simulink model "Atabey_Sim"  (R2025b)
settings: Solver=VariableStepAuto  StartTime=0.0  StopTime=simTime  RelTol=1e-3
undefined symbols (not defined in the file or in its folder): x0
libraries: aerolibfltsims x2, instrumentseriallib x2, slpidlib x1
settings Model: Creator=erayacikgz  LastModifiedBy=erayacikgz

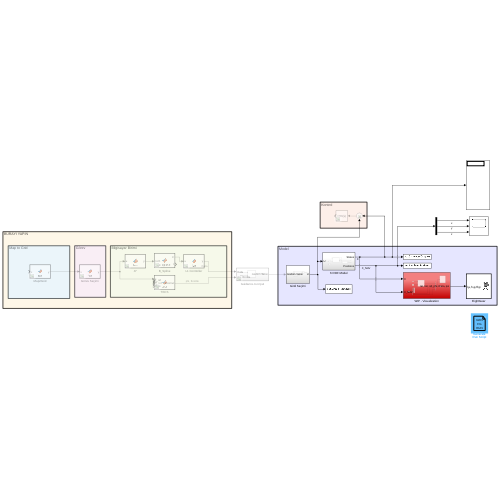
[thumbnail: Simulink's stored preview of the top-level diagram]
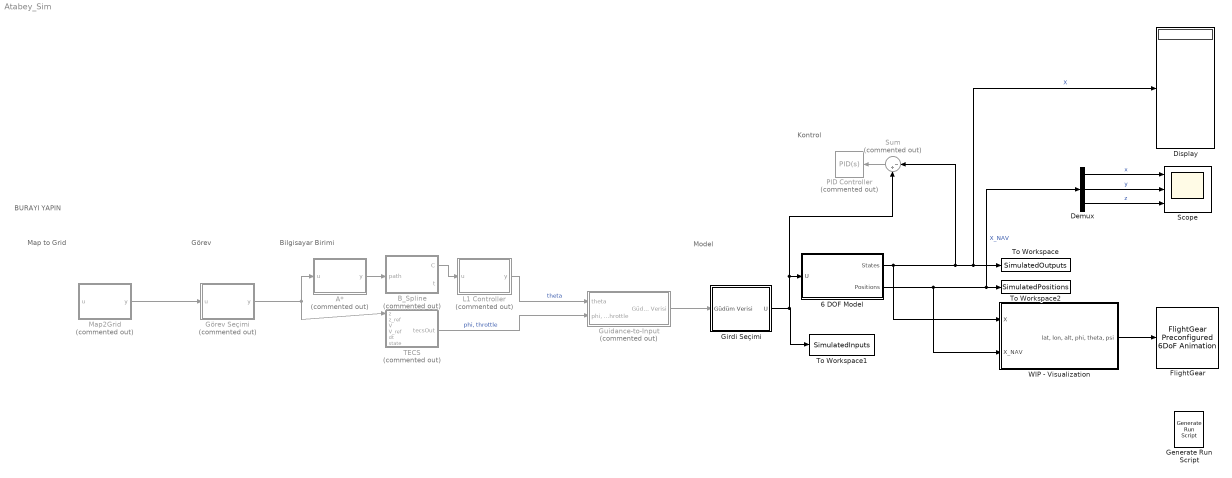
== system Atabey_Sim ==
  note: Görev
  note: BURAYI YAPIN
  note: Kontrol
  note: Map to Grid
  note: Bilgisayar Birimi
  note: Model
  6 DOF Model : Subsystem
  A* : MATLAB Function  Commented=on  TreatAsAtomicUnit=on
  B_Spline : MATLAB Function  Commented=on  TreatAsAtomicUnit=on
  Demux : Demux  Outputs=3
  Display : Display
  "FlightGear " : aerolibfltsims/FlightGear Preconfigured 6DoF Animation  xFlightGearVersion=v2019.1  DestinationIpAddress=127.0.0.1  DestinationPort=5502  SampleTime=1/30  packetVersion=24
  Generate Run Script : aerolibfltsims/Generate Run Script  Architecture=Linux  dataFlow=Send  GeometryModelName=HL20  AirportId=KSFO  RunwayId=10L  InitialAltitude=7224  InitialHeading=113  OffsetDistance=4.72  OffsetAzimuth=0  InstallScenery=off  DisableShaders=on  OriginAddress=127.0.0.1  DestinationPort=5502  OriginPort=5505  LocalAddress=127.0.0.1  OutputFileName=runfg.sh  FlightGearBaseDirectory=/usr/share/games/flightgear/
  Girdi Seçimi : Subsystem
  Guidance-to-Input : Subsystem  Commented=on
  Görev Seçimi : MATLAB Function  Commented=on  TreatAsAtomicUnit=on
  L1 Controller : MATLAB Function  Commented=on  TreatAsAtomicUnit=on
  Map2Grid : MATLAB Function  Commented=on  TreatAsAtomicUnit=on
  PID Controller : slpidlib/PID Controller  Commented=on  Controller=PID  Form=Parallel  TimeDomain=Continuous-time  UseExternalTs=off  SampleTime=-1  IntegratorMethod=Forward Euler  FilterMethod=Forward Euler  ControllerParametersSource=internal  P=1  I=1  UseKiTs=off  D=0  UseExternalDerivativeSource=off  N=100  UseFilter=on  TunerSelectOption=Transfer Function Based (PID Tuner App)  InitialConditionSource=internal  InitialConditionForIntegrator=0  InitialConditionForFilter=0  DifferentiatorICPrevScaledInput=0  ExternalReset=none  TrackingMode=off  Kt=1  LimitOutput=off  SatLimitsSource=internal  UpperSaturationLimit=inf  LowerSaturationLimit=-inf  LinearizeAsGain=on  AntiWindupMode=none  Kb=1  LimitIntegrator=off  UpperIntegratorSaturationLimit=inf  LowerIntegratorSaturationLimit=-inf  POutMin=[]  POutMax=[]  IOutMin=[]  IOutMax=[]  DOutMin=[]  DOutMax=[]  NOutMin=[]  NOutMax=[]  SumOutMin=[]  SumOutMax=[]  SaturationOutMin=[]  SaturationOutMax=[]  PParamMin=[]  PParamMax=[]  IParamMin=[]  IParamMax=[]  DParamMin=[]  DParamMax=[]  NParamMin=[]  NParamMax=[]  KbParamMin=[]  KbParamMax=[]  KtParamMin=[]  KtParamMax=[]  KbOutMin=[]  KbOutMax=[]  KtOutMin=[]  KtOutMax=[]  IntegratorOutMin=[]  IntegratorOutMax=[]  FilterOutMin=[]  FilterOutMax=[]  SumI1OutMin=[]  SumI1OutMax=[]  SumI2OutMin=[]  SumI2OutMax=[]  SumI3OutMin=[]  SumI3OutMax=[]  SumI4OutMin=[]  SumI4OutMax=[]  SumDOutMin=[]  SumDOutMax=[]  DifferentiatorOutMin=[]  DifferentiatorOutMax=[]  FilterDiffOutCoefMin=[]  FilterDiffOutCoefMax=[]  ReciprocalOutMin=[]  ReciprocalOutMax=[]  SumDenOutMin=[]  SumDenOutMax=[]  SumNumOutMin=[]  SumNumOutMax=[]  DivideOutMin=[]  DivideOutMax=[]  UdiffTsProdOutMin=[]  UdiffTsProdOutMax=[]  NTsProdOutMin=[]  NTsProdOutMax=[]  UintegralTsProdOutMin=[]  UintegralTsProdOutMax=[]  UngainTsProdOutMin=[]  UngainTsProdOutMax=[]  ClampingZeroOutDataTypeStr=Inherit: Inherit via back propagation  ClampingZeroOutMin=[]  ClampingZeroOutMax=[]  FilterDenConstantOutDataTypeStr=Inherit: Inherit via back propagation  FilterDenConstantOutMin=[]  FilterDenConstantOutMax=[]  PCopyOutDataTypeStr=Inherit: Inherit via back propagation  PCopyOutMin=[]  PCopyOutMax=[]  NCopyOutDataTypeStr=Inherit: Inherit via back propagation  NCopyOutMin=[]  NCopyOutMax=[]  IntegratorContinuousStateAttributes=''  IntegratorStateMustResolveToSignalObject=off  IntegratorRTWStateStorageClass=Auto  FilterContinuousStateAttributes=''  FilterStateMustResolveToSignalObject=off  FilterRTWStateStorageClass=Auto  ParallelPVariant=InternalParameters  IdealPVariant=Disabled  IVariant=InternalParameters  DVariant=InternalParameters  IntegratorVariant=Continuous  SatVariant=Disabled  AWVariant=Passthrough  PCopyVariant=Disabled  TRVariant=Disabled  FdbkBlocksVariant=Forward  IdealPFdbkVariant=Disabled  SatFdbkVariant=Disabled  DerivativeFilterVariant=ContFilter  NVariant=InternalParameters  NCopyVariant=Disabled  FilterICVariant=InternalICsFilter  IntegratorICVariant=InternalICs  ExternalResetVariant=Disabled  TRSumVariant=Passthrough  SumFdbkVariant=Disabled  SumVariant=Sum_PID  TsampFilterVariant=InternalTs  TsampNgainVariant=Passthrough  TsampIntegralVariant=Disabled_SignalSpec  ExternalSaturationOutDataTypeStr=Inherit: Same as second input  DerivativeSourceVariant=ErrorSignal  PreIntVariant=InternalPreInt
  Scope : Scope  NumInputPorts=3
      settings: ActiveDisplayYMinimum=-216.60563593004551  ActiveDisplayYMaximum=141.28895348469339
  Sum : Sum  Commented=on  Inputs=|-+
  TECS : MATLAB Function  Commented=on  TreatAsAtomicUnit=on
  To Workspace : ToWorkspace  VariableName=SimulatedOutputs  SaveFormat=Timeseries  SampleTime=-1
  To Workspace1 : ToWorkspace  VariableName=SimulatedInputs  SaveFormat=Timeseries  SampleTime=-1
  To Workspace2 : ToWorkspace  VariableName=SimulatedPositions  SaveFormat=Timeseries  SampleTime=-1
  WIP - Visualization : Subsystem
  wires:
  WIP - Visualization/1("lat, lon, alt, phi, theta, psi") -> "FlightGear "/1
  Map2Grid/1(y) -> Görev Seçimi/1(u)
  B_Spline/1(C) -> L1 Controller/1(u)
  A*/1(y) -> B_Spline/1(path)
  Guidance-to-Input/1(Güdüm Verisi) -> Girdi Seçimi/1(Güdüm Verisi)
  TECS/1(tecsOut) -> Guidance-to-Input/2("phi, throttle")  "phi, throttle"
  L1 Controller/1(y) -> Guidance-to-Input/1(theta)  "theta"
  6 DOF Model/2(Positions) -> Demux/1, To Workspace2/1, WIP - Visualization/2(X_NAV)  "X_NAV"
  6 DOF Model/1(States) -> Sum/1, Display/1, To Workspace/1, WIP - Visualization/1(X)  "X"
  Demux/1 -> Scope/1  "x"
  Demux/2 -> Scope/2  "y"
  Demux/3 -> Scope/3  "z"
  Görev Seçimi/1(y) -> TECS/1(z), A*/1(u)
  Girdi Seçimi/1(U) -> Sum/2, 6 DOF Model/1(U), To Workspace1/1
  Sum/1 -> PID Controller/1

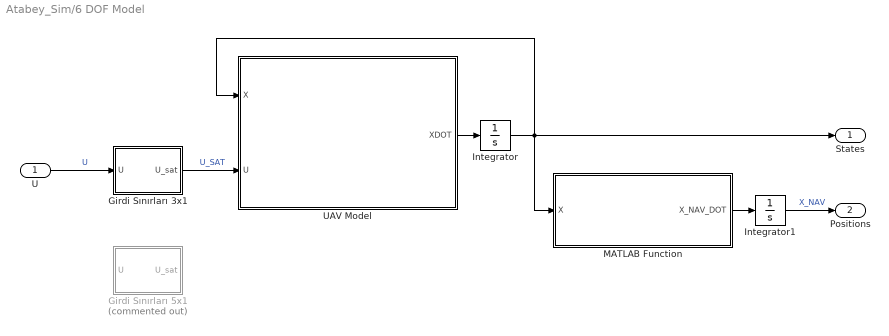
== system Atabey_Sim/6 DOF Model ==
  U : Inport
  Girdi Sınırları 3x1 : Subsystem
  Girdi Sınırları 5x1 : Subsystem  Commented=on
  Integrator : Integrator  InitialCondition=x0(:,:)
  Integrator1 : Integrator  InitialCondition=[0;0;0;]
  MATLAB Function : MATLAB Function  TreatAsAtomicUnit=on
  UAV Model : MATLAB Function  TreatAsAtomicUnit=on
  States : Outport
  Positions : Outport  Port=2
  wires:
  Girdi Sınırları 3x1/1(U_sat) -> UAV Model/2(U)  "U_SAT"
  Integrator1/1 -> Positions/1  "X_NAV"
  MATLAB Function/1(X_NAV_DOT) -> Integrator1/1
  Integrator/1 -> MATLAB Function/1(X), States/1, UAV Model/1(X)
  UAV Model/1(XDOT) -> Integrator/1
  U/1 -> Girdi Sınırları 3x1/1(U)  "U"

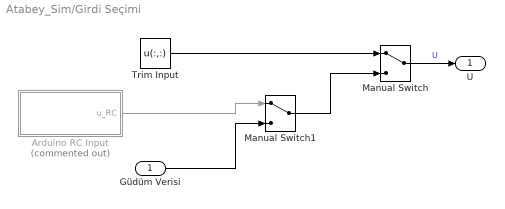
== system Atabey_Sim/Girdi Seçimi ==
  Güdüm Verisi : Inport
  Arduino RC Input : Subsystem  Commented=on
  Manual Switch : ManualSwitch
  Manual Switch1 : ManualSwitch
  Trim Input : Constant  Value=u(:,:)
  U : Outport
  wires:
  Güdüm Verisi/1 -> Manual Switch1/2
  Manual Switch/1 -> U/1  "U"
  Arduino RC Input/1(u_RC) -> Manual Switch1/1
  Manual Switch1/1 -> Manual Switch/2
  Trim Input/1 -> Manual Switch/1

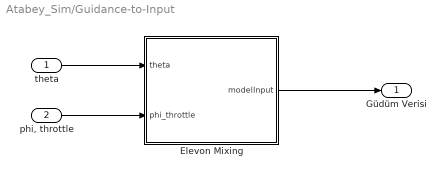
== system Atabey_Sim/Guidance-to-Input ==
  theta : Inport
  "phi, throttle" : Inport  Port=2
  Elevon Mixing : MATLAB Function  TreatAsAtomicUnit=on
  Güdüm Verisi : Outport
  wires:
  Elevon Mixing/1(modelInput) -> Güdüm Verisi/1
  "phi, throttle"/1 -> Elevon Mixing/2(phi_throttle)
  theta/1 -> Elevon Mixing/1(theta)

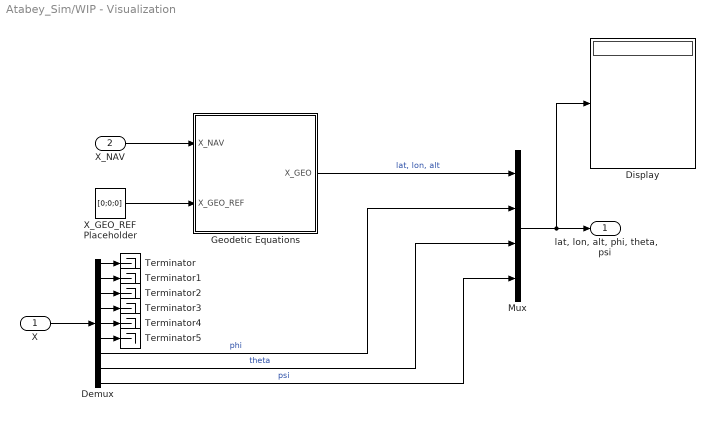
== system Atabey_Sim/WIP - Visualization ==
  X : Inport
  X_NAV : Inport  Port=2
  Demux : Demux  Outputs=9
  Display : Display
  Geodetic Equations : MATLAB Function  TreatAsAtomicUnit=on
  Mux : Mux
  Terminator{,1..5} (6 alike) : Terminator
  X_GEO_REF Placeholder : Constant  Value=[0;0;0]
  "lat, lon, alt, phi, theta, psi" : Outport
  wires:
  Mux/1 -> Display/1, "lat, lon, alt, phi, theta, psi"/1
  Geodetic Equations/1(X_GEO) -> Mux/1  "lat, lon, alt"
  Demux/9 -> Mux/4  "psi"
  Demux/7 -> Mux/2  "phi"
  X_NAV/1 -> Geodetic Equations/1(X_NAV)
  Demux/4 -> Terminator3/1
  X/1 -> Demux/1
  Demux/5 -> Terminator4/1
  X_GEO_REF Placeholder/1 -> Geodetic Equations/2(X_GEO_REF)
  Demux/8 -> Mux/3  "theta"
  Demux/3 -> Terminator2/1
  Demux/2 -> Terminator1/1
  Demux/1 -> Terminator/1
  Demux/6 -> Terminator5/1

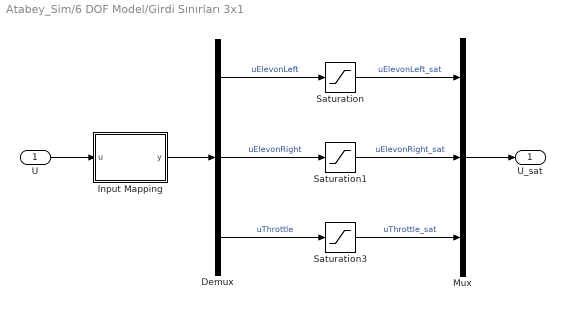
== system Atabey_Sim/6 DOF Model/Girdi Sınırları 3x1 ==
  U : Inport
  Demux : Demux  Outputs=3
  Input Mapping : MATLAB Function  TreatAsAtomicUnit=on
  Mux : Mux  Inputs=3
  Saturation : Saturate  UpperLimit=20  LowerLimit=-20
  Saturation1 : Saturate  UpperLimit=20  LowerLimit=-20
  Saturation3 : Saturate  UpperLimit=1  LowerLimit=0
  U_sat : Outport
  wires:
  Saturation3/1 -> Mux/3  "uThrottle_sat"
  Demux/3 -> Saturation3/1  "uThrottle"
  Saturation1/1 -> Mux/2  "uElevonRight_sat"
  Demux/1 -> Saturation/1  "uElevonLeft"
  U/1 -> Input Mapping/1(u)
  Saturation/1 -> Mux/1  "uElevonLeft_sat"
  Demux/2 -> Saturation1/1  "uElevonRight"
  Mux/1 -> U_sat/1
  Input Mapping/1(y) -> Demux/1

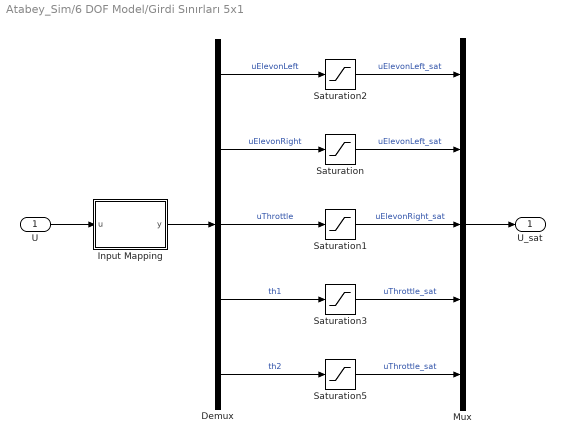
== system Atabey_Sim/6 DOF Model/Girdi Sınırları 5x1 ==
  U : Inport
  Demux : Demux  Outputs=5
  Input Mapping : MATLAB Function  TreatAsAtomicUnit=on
  Mux : Mux  Inputs=5
  Saturation : Saturate  UpperLimit=20  LowerLimit=-20
  Saturation1 : Saturate  UpperLimit=20  LowerLimit=-20
  Saturation2 : Saturate  UpperLimit=20  LowerLimit=-20
  Saturation3 : Saturate  UpperLimit=1  LowerLimit=0
  Saturation5 : Saturate  UpperLimit=1  LowerLimit=0
  U_sat : Outport
  wires:
  U/1 -> Input Mapping/1(u)
  Mux/1 -> U_sat/1
  Input Mapping/1(y) -> Demux/1
  Demux/1 -> Saturation2/1  "uElevonLeft"
  Demux/2 -> Saturation/1  "uElevonRight"
  Demux/3 -> Saturation1/1  "uThrottle"
  Demux/4 -> Saturation3/1  "th1"
  Demux/5 -> Saturation5/1  "th2"
  Saturation2/1 -> Mux/1  "uElevonLeft_sat"
  Saturation/1 -> Mux/2  "uElevonLeft_sat"
  Saturation1/1 -> Mux/3  "uElevonRight_sat"
  Saturation3/1 -> Mux/4  "uThrottle_sat"
  Saturation5/1 -> Mux/5  "uThrottle_sat"

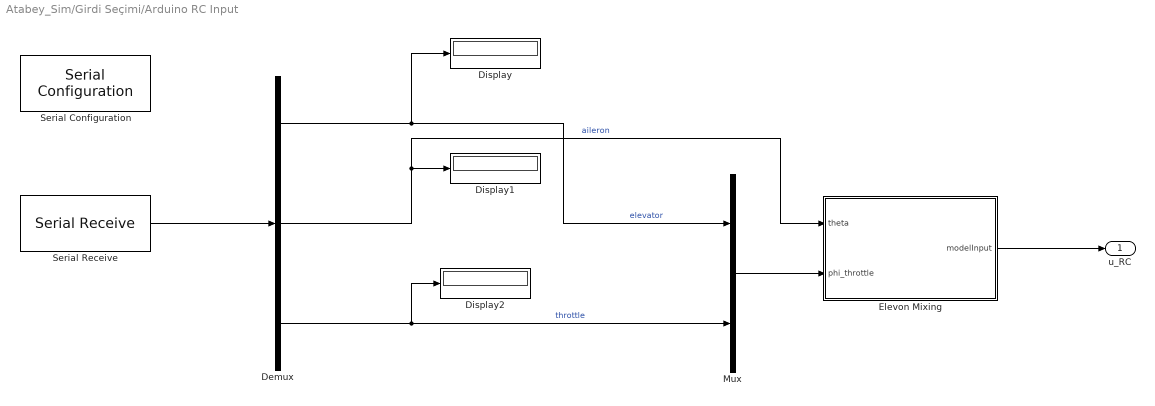
== system Atabey_Sim/Girdi Seçimi/Arduino RC Input ==
  Demux : Demux  Outputs=3
  Display : Display
  Display1 : Display
  Display2 : Display
  Elevon Mixing : MATLAB Function  TreatAsAtomicUnit=on
  Mux : Mux  Inputs=2
  Serial Configuration : instrumentseriallib/Serial Configuration  Priority=-200000  PortSel=/dev/ttyUSB0  Port=/dev/ttyUSB0  ComPort=/dev/ttyUSB0  BaudRate=9600  DataBits=8  Parity=none  StopBits=1  ByteOrder=little-endian  FlowControl=none  Timeout=10  SimulateUsing=Interpreted execution  BlockInModel=on  aMode=1
      settings: LibrarySourceBlock=c2000lib/Host Communication/Serial Configuration
  Serial Receive : instrumentseriallib/Serial Receive  Priority=1  PortSel=/dev/ttyUSB0  Port=/dev/ttyUSB0  ComPort=/dev/ttyUSB0  DataType=int16  SaveDataType=uint8  ToggleHeader=on  Header=[255]  ToggleDataSize=on  DataSize=[1 3]  ToggleTerminator=off  Terminator=<none>  CustomTerminator=[]  InputFormat=Column major  EnableBlockingMode=on  ActionDataUnavailable=Output last received value  ActionWhenDataUnavailable=Output last received value  CustomValue=0  SampleTime=0.01  SimulateUsing=Interpreted execution  BlockInModel=on  aMode=1  LibraryInUse=c2000lib
      settings: LibrarySourceBlock=c2000lib/Host Communication/Serial Receive
  u_RC : Outport
  wires:
  Serial Receive/1 -> Demux/1
  Demux/3 -> Display2/1, Mux/2  "throttle"
  Demux/1 -> Mux/1, Display/1  "elevator"
  Demux/2 -> Elevon Mixing/1(theta), Display1/1  "aileron"
  Elevon Mixing/1(modelInput) -> u_RC/1
  Mux/1 -> Elevon Mixing/2(phi_throttle)

== matlab function Atabey_Sim/Map2Grid ==
  data: u input; y output
function y = fcn(u)

y = u;

== matlab function Atabey_Sim/Görev Seçimi ==
  data: u input; y output
function y = fcn(u)

y = u;

== matlab function Atabey_Sim/6 DOF Model/MATLAB Function ==
  data: X input; X_NAV_DOT output
function X_NAV_DOT  = NavigationEquations(X)

P_N_dot = X(1)*cos(X(8))*cos(X(9))...
    + X(2)*(-cos(X(7))*sin(X(9)) + sin(X(7))*sin(X(8))*cos(X(9)))...
    + X(3)*(sin(X(7))*sin(X(9)) + cos(X(7))*sin(X(8))*cos(X(9)));

P_E_dot = X(1)*cos(X(8))*sin(X(9))...
    + X(2)*(cos(X(7))*cos(X(9)) + sin(X(7))*sin(X(8))*sin(X(9)))...
    + X(3)*(-sin(X(7))*cos(X(9)) + cos(X(7))*sin(X(8))*sin(X(9)));

h_dot = X(1)*sin(X(8)) - X(2)*sin(X(7))*cos(X(8)) - X(3)*cos(X(7))*cos(X(8));

X_NAV_DOT = [P_N_dot;
             P_E_dot;
             h_dot];

end

== matlab function Atabey_Sim/6 DOF Model/UAV Model ==
  data: X input double size=[9 1]; XDOT output double size=[9 1]; U input double
% MATLAB/ATABEY_dynamics
% Fonksiyon, dinamik dosyasını çağırır, modüler değişiklik yapmak için

function XDOT = ATABEY_model(X, U)

    XDOT = ATABEY_dynamics(X, U);

end

== matlab function Atabey_Sim/WIP - Visualization/Geodetic Equations ==
  data: X_NAV input; X_GEO output; X_GEO_REF input
function X_GEO = FlatEarthtoGeodetic(X_NAV, X_GEO_REF)

PN = X_NAV(1);               % Kuzey (m)
PE = X_NAV(2);               % Doğu  (m)
PH = X_NAV(3);               % Positive Down

lat0 = X_GEO_REF(1);
lon0 = X_GEO_REF(2);
alt0 = X_GEO_REF(3);

% WGS-84
a = 6378137.0;               % Semi-major axis (m)
f = 1/298.257223563;         % Flattening
e2 = 2*f - f^2;              % Eccentricity squared

lat0_rad = deg2rad(lat0);

% Eğri Yarıçapı, Prime Vertical
N = a / sqrt(1 - e2 * sin(lat0_rad)^2);

% Eğri Yarıçapı, Meridyen
M = a * (1 - e2) / (1 - e2 * sin(lat0_rad)^2)^1.5;

% PN/PE -> delta lat/lon (rad)
d_lat = PN / M;
d_lon = PE / (N * cos(lat0_rad));

% Çıktı
lat = lat0 + rad2deg(d_lat); % deg
lon = lon0 + rad2deg(d_lon); % deg
alt = -1*(alt0 - PH);             % m

X_GEO = [lat,lon,alt];

end

== matlab function Atabey_Sim/A* ==
  data: u input; y output
function y = fcn(u)

y = u;

== matlab function Atabey_Sim/B_Spline ==
  data: path input; C output; t output
function [C, t] = B_Spline(path)
% Inputs:
%   path - A* result [n x 2] or [n x 3] of [row, col] grid indices
k = 4;      % Spline order (degree = k-1). Default: 4 (cubic)
n = 500;    % Number of output curve points. Default: 500
%
% Outputs:
%   C    - Evaluated curve points [n x d]  <-- feed this to L1
  % t    - Parameter values [1 x n]

% Defaults
if nargin < 2, k = 4;   end
if nargin < 3, n = 500; end

%% A* -> Control Points
P = double(path);

if iscolumn(P) && size(P, 2) == 1
    error('path_to_bspline: path must be [n x 2] or [n x 3], not a linear index vector.');
end

% Remove consecutive duplicates (prevents zero-length knot spans)
mask = [true; any(diff(P, 1, 1) ~= 0, 2)];
P    = P(mask, :);

% [row, col] -> [x, y]  (comment out if A* already returns [x, y])
P = fliplr(P);

%% Evaluate B-Spline
[m, d]    = size(P);
num_knots = m + k;

% Clamped uniform knot vector
knots = [zeros(1, k), linspace(0, 1, num_knots - 2*k + 2), ones(1, k)];

t = linspace(knots(k), knots(m + 1), n);
C = zeros(n, d);

for i = 1:n
    % de Boor evaluation at t(i)
    ti = t(i);

    % Knot span index
    if ti == knots(end)
        r = m;
    else
        r = min(find(knots <= ti, 1, 'last') - 1, m);
    end

    % Local control points for this span
    idx = max(1, min((r - k + 1):r, m));
    dp  = P(idx, :);

    % de Boor recursion
    for s = 1:(k - 1)
        for j = k:-1:(s + 1)
            i_knot = r - k + j;
            denom  = knots(i_knot + k - s) - knots(i_knot);
            alpha  = 0;
            if denom ~= 0
                alpha = (ti - knots(i_knot)) / denom;
            end
            dp(j, :) = (1 - alpha) * dp(j - 1, :) + alpha * dp(j, :);
        end
    end

    C(i, :) = dp(k, :);
end

end

== matlab function Atabey_Sim/L1 Controller ==
  data: u input; y output
function y = fcn(u)

y = u;

== matlab function Atabey_Sim/TECS ==
  data: z input; tecsOut output; z_ref input; V input; V_ref input; dt input; state input
function tecsOut = tecs(z, z_ref, V, V_ref, dt, state)
%   Inputs:
%     z      - Current altitude        (m)
%     z_ref  - Desired altitude        (m)
%     V      - Current airspeed        (m/s)
%     V_ref  - Desired airspeed        (m/s)
%     dt     - Timestep                (s)
%     state  - Persistent integrator state (struct, init with tecs_init())
%
%   Outputs:
%     theta_cmd - Pitch angle command  (rad)
%     throttle  - Throttle command     [0, 1]
%
%   Note: outputs theta (pitch), not phi (roll).
%         Feed theta_cmd into function_to_model() as theta.

    g = 9.81;

    % --- Gains (tune for your airframe) ---
    K_thr_E    = 0.5;   % Throttle proportional gain (total energy)
    K_thr_Edot = 1.0;   % Throttle derivative gain   (energy rate)
    K_thr_I    = 0.1;   % Throttle integral gain
    K_pit_L    = 0.5;   % Pitch proportional gain     (energy balance)
    K_pit_Ldot = 1.0;   % Pitch derivative gain
    K_pit_I    = 0.05;  % Pitch integral gain

    throttle_min = 0.0;
    throttle_max = 1.0;
    theta_min    = deg2rad(-20);
    theta_max    = deg2rad(20);

    % --- Specific energy (normalised by mass*g) ---
    E_kin     = 0.5 * V^2     / g;
    E_kin_ref = 0.5 * V_ref^2 / g;

    E_pot     = z;
    E_pot_ref = z_ref;

    % Total specific energy
    E     = E_kin     + E_pot;
    E_ref = E_kin_ref + E_pot_ref;

    % Energy balance (distribution): positive = more altitude, less speed
    L     = E_pot     - E_kin;
    L_ref = E_pot_ref - E_kin_ref;

    % --- Errors ---
    E_err = E_ref - E;
    L_err = L_ref - L;

    % --- Error rates (finite difference) ---
    E_err_dot = (E_err - state.E_err_prev) / dt;
    L_err_dot = (L_err - state.L_err_prev) / dt;

    % --- Integrators ---
    E_int = state.E_int + E_err * dt;
    L_int = state.L_int + L_err * dt;

    % --- Control outputs ---
    throttle  = K_thr_E * E_err + K_thr_Edot * E_err_dot + K_thr_I * E_int;
    theta_cmd = K_pit_L * L_err + K_pit_Ldot * L_err_dot + K_pit_I * L_int;

    % --- Clamp outputs ---
    throttle  = max(throttle_min, min(throttle_max, throttle));
    theta_cmd = max(theta_min,    min(theta_max,    theta_cmd));

    % --- Update state (return for next call) ---
    state.E_err_prev = E_err;
    state.L_err_prev = L_err;
    state.E_int      = E_int;
    state.L_int      = L_int;

end


function state = tecs_init()
% TECS_INIT  Initialise integrator state for TECS.
    state.E_err_prev = 0;
    state.L_err_prev = 0;
    state.E_int      = 0;
    state.L_int      = 0;
end

== matlab function Atabey_Sim/Guidance-to-Input/Elevon Mixing ==
  data: theta input; modelInput output; phi_throttle input
function modelInput  = elevonMix(theta, phi_throttle)
    phi = phi_throttle(1);
    
    % Elevon mixing
    elevon_left  = theta + phi;
    elevon_right = theta - phi;

    % % Clamp to actuator limits 
    % -> Gerek yok gibi?
    % elevon_left  = max(-1.0, min(1.0, elevon_left));
    % elevon_right = max(-1.0, min(1.0, elevon_right));

    % Throttle passthrough
    throttle_out = phi_throttle(2);

    modelInput = [elevon_left;elevon_right;throttle_out];

end

== matlab function Atabey_Sim/Girdi Seçimi/Arduino RC Input/Elevon Mixing ==
  data: theta input; modelInput output; phi_throttle input
function modelInput  = elevonMix(theta, phi_throttle)
    phi = phi_throttle(1);
    
    % Elevon mixing
    elevon_left  = theta + phi;
    elevon_right = theta - phi;

    % % Clamp to actuator limits 
    % -> Gerek yok gibi?
    % elevon_left  = max(-1.0, min(1.0, elevon_left));
    % elevon_right = max(-1.0, min(1.0, elevon_right));

    % Throttle passthrough
    throttle_out = phi_throttle(2);

    modelInput = [elevon_left;elevon_right;throttle_out];

end

== matlab function Atabey_Sim/6 DOF Model/Girdi Sınırları 3x1/Input Mapping ==
  data: u input; y output
function y = fcn(u)

% Map first two values from [-100, 100] to [-20, 20]
y1 = double(u(1)) * (20 / 100);
y2 = double(u(2)) * (20 / 100);

% Map last value from [0, 100] to [0, 1]
y3 = double(u(end)) * (1 / 100);

y = [y1; y2; y3];

== matlab function Atabey_Sim/6 DOF Model/Girdi Sınırları 5x1/Input Mapping ==
  data: u input; y output
function y = fcn(u)

% Map first two values from [-100, 100] to [-20, 20]
y1 = double(u(1)) * (20 / 100);
y2 = double(u(2)) * (20 / 100);

% Map last value from [0, 100] to [0, 1]
y3 = double(u(end)) * (1 / 100);

y = [y1; y2; y3];
